simulink model "controller_final"  (R2022b)
settings: Solver=ode4  StartTime=0.0  StopTime=2  FixedStep=0.001  RelTol=1e-3  EnableMultiTasking=on
settings Model: Creator=hjy34  LastModifiedBy=dlrbg

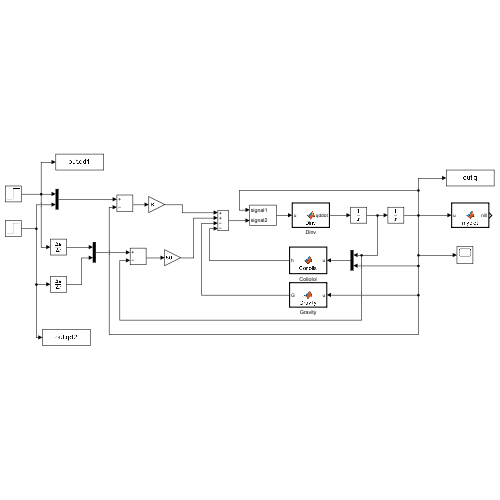
[thumbnail: Simulink's stored preview of the top-level diagram]
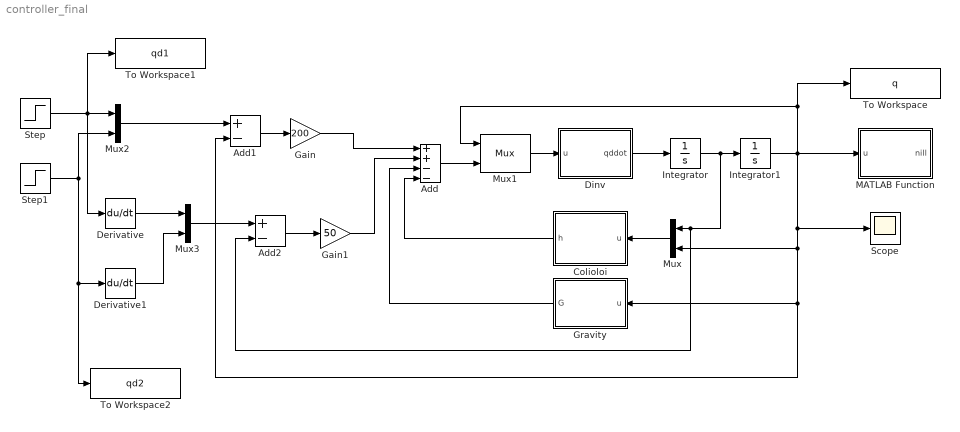
== system controller_final ==
  Add : Sum  Inputs=++--
  Add1 : Sum  Inputs=+-
  Add2 : Sum  Inputs=+-
  Colioloi : MATLAB Function  TreatAsAtomicUnit=on
  Derivative : Derivative
  Derivative1 : Derivative
  Dinv : MATLAB Function  TreatAsAtomicUnit=on
  Gain : Gain  Gain=200
  Gain1 : Gain  Gain=50
  Gravity : MATLAB Function  TreatAsAtomicUnit=on
  Integrator : Integrator  InitialCondition=[0 0]'
  Integrator1 : Integrator  InitialCondition=[-0.4538 -0.4538]'
  MATLAB Function : MATLAB Function  TreatAsAtomicUnit=on
  Mux{,1..3} (4 alike) : Mux  Inputs=2
      Mux1 settings: DisplayOption=signals
  Scope : Scope
  Step : Step  Time=2  SampleTime=0
  Step1 : Step  Time=2  SampleTime=0  VectorParams1D=off
  To Workspace : ToWorkspace  VariableName=q  SaveFormat=Timeseries  SampleTime=-1
  To Workspace1 : ToWorkspace  VariableName=qd1  SaveFormat=Timeseries  SampleTime=-1
  To Workspace2 : ToWorkspace  VariableName=qd2  SaveFormat=Timeseries  SampleTime=-1
  wires:
  Dinv/1(qddot) -> Integrator/1
  Integrator/1 -> Add2/2, Mux/1, Integrator1/1
  Mux/1 -> Colioloi/1(u)
  Add1/1 -> Gain/1
  Add/1 -> Mux1/2
  Mux1/1 -> Dinv/1(u)
  Integrator1/1 -> Gravity/1(u), Add1/2, Mux/2, Scope/1, Mux1/1, To Workspace/1, MATLAB Function/1(u)
  Step/1 -> Derivative/1, Mux2/1, To Workspace1/1
  Mux2/1 -> Add1/1
  Step1/1 -> To Workspace2/1, Derivative1/1, Mux2/2
  Derivative/1 -> Mux3/1
  Derivative1/1 -> Mux3/2
  Mux3/1 -> Add2/1
  Add2/1 -> Gain1/1
  Gain1/1 -> Add/2
  Gain/1 -> Add/1
  Colioloi/1(h) -> Add/4
  Gravity/1(G) -> Add/3

== matlab function controller_final/Dinv ==
  data: u input; qddot output
function qddot = Dinv(u)
m1=1;m2=1;l1=0.4;l2=0.4;
q1=u(1);q2=u(2);
d11=(m1+m2)*l1^2 + m2*l2^2 + 2*m2*l1*l2*cos(q2);
d12=m2*l2^2 + m2*l1*l2*cos(q2);
d21=m2*l2^2 + m2*l1*l2*cos(q2);
d22=m2*l2^2;
D=[d11 d12;d21 d22];
D_inv = inv(D);
C_input=[u(3);u(4)];
qddot = ((D_inv) * C_input);

== matlab function controller_final/Colioloi ==
  data: u input; h output
function h = Coriolis(u)
dotq1=u(1);dotq2=u(2);q1=u(3);q2=u(4);
m1=5;m2=5;l1=0.4;l2=0.4;
h1=-m2*l1*l2*sin(q2)*(2*dotq1*dotq2+dotq2^2);
h2=m2*l1*l2*dotq1^2*sin(q2);
h = [h1;h2];

== matlab function controller_final/MATLAB Function ==
  data: u input; nill output
function nill = myplot(u)
q1=u(1);q2=u(2);
x1=cos(q1);
y1=sin(q1);
x2=x1+cos(q1+q2);
y2=y1+sin(q1+q2);
plot([0 x1 x2],[0 y1 y2]);
axis([-2 2 0 2]);
nill=0;

== matlab function controller_final/Gravity ==
  data: u input; G output
function G = Gravity(u)
m1=5;m2=5;l1=0.4;l2=0.4;g=9.8;
q1=u(1);q2=u(2);
G1=(m1+m2)*g*l1*cos(q1) + m2*g*l2*cos(q1+q2);
G2=m2*g*l2*cos(q1+q2);
G=[G1;G2];
